simulink model "Sixphase_PMSM_doubleDQ"  (R2023b)
settings: Solver=ode23t  StartTime=0.0  StopTime=0.5  MaxStep=1e-4  RelTol=1e-3  EnableMultiTasking=on
InitFcn:
  | Ts = 1e-6;
undefined symbols (not defined in the file): powergui, sps_lib
libraries: powerlib_extras x7, spsVoltageMeasurementLib x4, spsUniversalBridgeLib x2, spsDCVoltageSourceLib x1
settings Model: Creator=y  LastModifiedBy=Guoguo
settings SolverCC: AlgebraicLoopSolver=TrustRegion
settings DataIOCC: LimitDataPoints=on  SaveFormat=Array  SignalLoggingSaveFormat=ModelDataLogs  ReturnWorkspaceOutputs=off
settings OptimizationCC: ExpressionDepthLimit=2147483647  InitFltsAndDblsToZero=on  LifeSpan=inf
settings DebuggingCC: SaveWithParameterizedLinksMsg=none  UnderspecifiedInitializationDetection=Classic  MergeDetectMultiDrivingBlocksExec=none  SignalResolutionControl=TryResolveAllWithWarning  SolverPrmCheckMsg=warning  MultiTaskDSMMsg=warning  MultiTaskCondExecSysMsg=none  FcnCallInpInsideContextMsg=warning  UnconnectedInputMsg=warning  UnconnectedOutputMsg=warning  UnconnectedLineMsg=warning  StateNameClashWarn=warning  SFUnexpectedBacktrackingDiag=warning  SFNoUnconditionalDefaultTransitionDiag=warning  SFExecutionAtInitializationDiag=none  ArithmeticOperatorsInVariantConditions=warning
settings HardwareCC: ProdBitPerPointer=32  ProdBitPerSizeT=32  ProdBitPerPtrDiffT=32  ProdLargestAtomicFloat=None  ProdIntDivRoundTo=Undefined  ProdEndianess=Unspecified  ProdWordSize=32  ProdHWDeviceType=32-bit Generic
settings ModelReferenceCC: PropagateSignalLabelsOutOfModel=off
settings SFSimCC: SimUseLocalCustomCode=off  CustomCodeUndefinedFunction=UseInterfaceOnly
settings RTWCC: RTWUseLocalCustomCode=off
settings CodeAppCC: StateflowObjectComments=on
settings GRTTargetCC: TargetFcnLib=ansi_tfl_tmw.mat  TargetLangStandard=C89/C90 (ANSI)  CombineOutputUpdateFcns=off  GRTInterface=on
settings ConfigComp: CovMetricSettings=dw  CovSaveCumulativeToWorkspaceVar=on  CovSaveSingleToWorkspaceVar=on  CovExternalEMLEnable=off  CovSFcnEnable=off
settings SimscapeCC: SimscapeNormalizeSystem=off

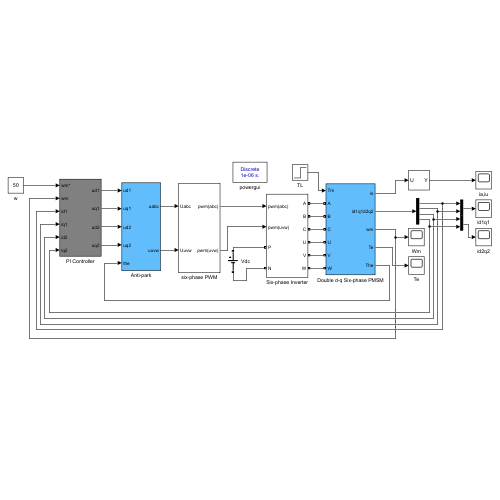
[thumbnail: Simulink's stored preview of the top-level diagram]
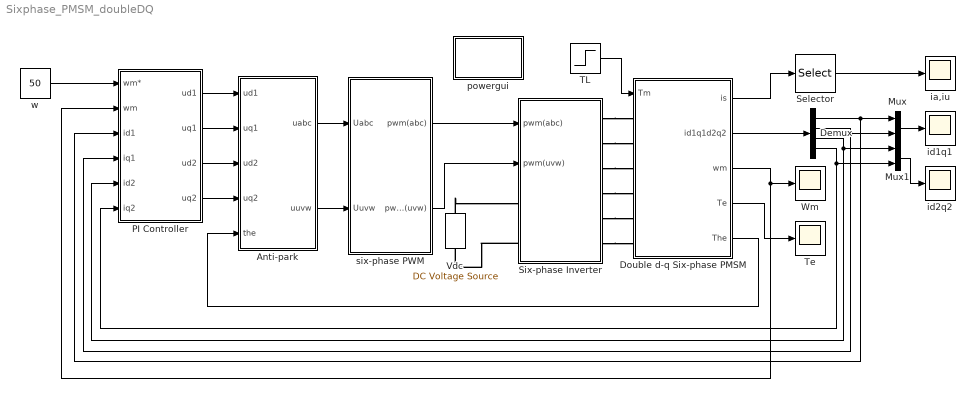
== system Sixphase_PMSM_doubleDQ ==
  Anti-park : Subsystem
  Demux : Demux
  Double d-q Six-phase PMSM : Subsystem  mask{R=1.4, Ld=4.85e-3, Lq=4.85e-3, Ldd=3.15e-3, Lqq=3.15e-3, p=3, Flux=0.68, J=0.015, F=0}
  Mux : Mux  Inputs=2
  Mux1 : Mux  Inputs=2
  PI Controller : Subsystem
  Selector : Selector  InputPortWidth=6  IndexOptions=Index vector (dialog)  Indices=[1 4]  OutputSizes=1
  Six-phase Inverter : Subsystem
  TL : Step  Time=0.2  After=50  SampleTime=0
  Te : Scope
  Vdc : spsDCVoltageSourceLib/DC Voltage Source  Amplitude=300  Measurements=None
  Wm : Scope
  ia,iu : Scope
  id1q1 : Scope
  id2q2 : Scope
  powergui : Subsystem  Priority=1  AncestorBlock=sps_lib/powergui  InitFcn=powergui( 'InitFcn_Callback' , gcb , 0 , [ ] );  mask(PSB option menu block){SimulationMode=Discrete, SampleTime=1e-6, frequency=60, Iterations=50, frequencyindice=0, Pbase=100e6, ErrMax=1e-4, UnitsV=kV, UnitsW=MW, buscounter=0, FunctionMessages=off, echomessages=off, EnableUseOfTLC=off, CurrentSourceSwitches=on, DisableSnubberDevices=off, DisableRonSwitches=off, DisableVfSwitches=off, DisplayEquations=off, AutomaticDiscreteSolvers=off, SolverType=Tustin/Backward Euler (TBE), Interpol=off, ExternalGateDelay=off, methode=off, Ts=100, x0status=blocks, SPID=off, SwTol=0, HookPort=off, NonlinearTolerance=1e-4, nMaxIteration=100, ContinueOnMaxIteration=off, RestoreLinks=warning, ResistiveCurrentMeasurement=off, Frange=[0:2:500], Ylog=off, Xlog=on, ShowGrid=off, save=off, variable=ZData, structure=0, ZoomFFT=off, StartTime=0.0, cycles=1, DisplayStyle=1, fundamental=60, FreqAxis=off, MaxFrequency=1000, frequencyindicesteady=1, RmsSteady=1, display=off}
      mask prompts: SimulationMode "Simulation type:"; SampleTime "Sample time (s):"; frequency "Frequency (Hz):"; Iterations "Max iterations"; frequencyindice "Frequency (Hz)"; Pbase "Base power (VA)"; ErrMax "PQ tolerance (pu)"; UnitsV "Voltage units"; UnitsW "Power units"; buscounter "Load flow bus counter"; FunctionMessages "Disable Specialized Power Systems warnings"; echomessages "Display Specialized Power Systems compilation messages"; EnableUseOfTLC "Use TLC file when in Accelerator Simulation Mode and for code generation"; CurrentSourceSwitches "Disable ideal switching"; DisableSnubberDevices "Disable snubbers in switching devices"; DisableRonSwitches "Disable Ron resistances in switching devices"; DisableVfSwitches "Disable forward voltages in switching devices"; DisplayEquations "Display circuit differential equations"; AutomaticDiscreteSolvers "Automatically handle Discrete solver and Advanced tab solver settings of blocks"; SolverType "Discrete solver"; Interpol "Interpolate switching events"; ExternalGateDelay "Use time-stamped gate signals"; methode "Store switching topologies"; Ts "Buffer size (MBytes):"; x0status "Start simulation with initial electrical states from:"; SPID "Use ideal switching devices"; SwTol "Switch tolerance"; HookPort "Allow multiple powergui blocks"; NonlinearTolerance "Solver tolerance"; nMaxIteration "Maximum number of iterations"; ContinueOnMaxIteration "Continue Simulation if maximum number of iterations is reached"; RestoreLinks "Restore disabled links of Simscape Power Systems ST blocks:"; ResistiveCurrentMeasurement "Use non ideal current measurement blocks (1e-4Ohm internal resistance)"; Frange "Frequency Range"; Ylog "Log impedance"; Xlog "log Frequency"; ShowGrid "grid"; save "Save Data To Workspace"; variable "Variable Name"; structure "Structure Name (PSBFFTSCOPE)"; ZoomFFT "ZoomFFT (PSBFFTSCOPE)"; StartTime "Start Time (PSBFFTSCOPE)"; cycles "Cycles (PSBFFTSCOPE)"; DisplayStyle "Display style (PSBFFTSCOPE)"; fundamental "Fundamental (PSBFFTSCOPE)"; FreqAxis "Frequency Axis (PSBFFTSCOPE)"; MaxFrequency "Max Frequency (PSBFFTSCOPE)"; frequencyindicesteady "Frequency indice (STEADYSTATE)"; RmsSteady "RMS display (STEADYSTATE)"; display "Display Results"
      mask help: Set simulation type, simulation parameters, and preferences.
      mask init:
      | dispMessage = '';
      | dispMessage = powergui('MaskInitialization',gcb,SimulationMode,SampleTime);
      settings: LibrarySourceBlock=sps_lib/powergui  PreSaveFcn=powergui( 'PreSaveFcn_Callback' , gcb , [ ] , [ ] );  OpenFcn=sps_rtmsupport('OpenFcn',gcbh)
      mask Help: helpview(psbhelp)
      mask TypeOptions SimulationMode: Continuous | Discrete | Phasor | Discrete phasor
      mask Callback SimulationMode: powergui('SimulationType',[],[],gcb);
      mask TypeOptions UnitsV: V | kV
      mask TypeOptions UnitsW: W | kW | MW
      mask Callback CurrentSourceSwitches: powergui('SimulationType',[],[],gcb);
      mask Callback AutomaticDiscreteSolvers: powergui('SimulationType',[],[],gcb);
      mask TypeOptions SolverType: Tustin/Backward Euler (TBE) | Tustin | Backward Euler
      mask Callback SolverType: powergui('SimulationType',[],[],gcb);
      mask Callback Interpol: powergui('SimulationType',[],[],gcb);
      mask Callback ExternalGateDelay: powergui('SimulationType',[],[],gcb);
      mask Callback methode: powergui('SimulationType',[],[],gcb);
      mask TypeOptions x0status: blocks | steady | zero
      mask TypeOptions RestoreLinks: yes | warning | no
      mask Callback display: sps_rtmsupport('parametereditingmodes',gcbh) % Will be executed last in parameter callbacks to ensure mask enable consistency
      mask DialogControl SolverTab Prompt: Solver
      mask DialogControl AutoSolverNote Prompt: The Simulation type parameter is governed by Simulink. To access the Powergui solver settings, unselect auto (Automatic solver selection) solver in the Simulink solver options.
      mask DialogControl Apps Prompt: Apps
      mask DialogControl StateAnalyzer Prompt: Measurements and States Analyzer
      mask DialogControl StateAnalyzer Callback: powerStates(bdroot(gcb))
      mask DialogControl LineParameterCalculator Prompt: Line Parameter Calculator
      mask DialogControl LineParameterCalculator Callback:
      | close_system(gcb)
      | powerLineParameters
      mask DialogControl CableParameterCalculator Prompt: Cable Parameter Calculator
      mask DialogControl CableParameterCalculator Callback:
      | close_system(gcb)
      | powerCableParameters
      mask DialogControl LineDecoupler Prompt: Line Decoupler
      mask DialogControl LineDecoupler Tooltip: Click to replace selected Distributed Parameters Line blocks with Decoupling Line blocks
      mask DialogControl LineDecoupler Callback:
      | close_system(gcb);
      | DecouplingLineReplace(gcs)
      mask DialogControl LoadFlowAnalyzer Prompt: Load Flow Analyzer
      mask DialogControl LoadFlowAnalyzer Callback:
      | close_system(gcb)
      | powerLoadFlow
      mask DialogControl LoadFlowParameters Prompt: Load Flow Parameters
      mask DialogControl ImpedanceCalculator Prompt: Impedance Calculator
      mask DialogControl ImpedanceCalculator Callback:
      | close_system(gcb);
      | powerImpedance(bdroot(gcs));
      mask DialogControl FFTAnalyzer Prompt: FFT Analyzer
      mask DialogControl FFTAnalyzer Callback:
      | close_system(gcb)
      | power_fftscope(bdroot(gcb),gcb)
      mask DialogControl LinearSystemAnalyzer Prompt: Linear System Analyzer
      mask DialogControl LinearSystemAnalyzer Callback:
      | close_system(gcb)
      | power_ltiview(bdroot(gcb))
      mask DialogControl HysteresisDesigner Prompt: Hysteresis Designer
      mask DialogControl HysteresisDesigner Callback:
      | close_system(gcb)
      | powerHysteresis('hysteresis.mat')
      mask DialogControl BlockCustomizer Prompt: Block Customizer
      mask DialogControl BlockCustomizer Callback:
      | close_system(gcb);
      | power_customize;
      mask DialogControl ReportGenerator Prompt: Report Generator
      mask DialogControl ReportGenerator Callback:
      | close_system(gcb)
      | power_report(bdroot(gcb))
      mask DialogControl obsolete Prompt: ...
      mask DialogControl MachineInitialization Prompt: Machine Initialization
      mask DialogControl MachineInitialization Callback:
      | close_system(gcb)
      | powericon('machineInitTool',bdroot(gcb),gcb)
      mask DialogControl Preferences Prompt: Preferences
      mask DialogControl Solver Prompt: Solver
      mask DialogControl SolverDetails Prompt: Solver details for nonlinear elements
      mask Display: color('blue'),disp(dispMessage)
  six-phase PWM : Subsystem
  w : Constant  Value=50
  wires:
  Double d-q Six-phase PMSM/2(id1q1d2q2) -> Demux/1
  Demux/1 -> Mux/1, PI Controller/3(id1)
  Demux/2 -> Mux/2, PI Controller/4(iq1)
  Demux/3 -> Mux1/1, PI Controller/5(id2)
  Demux/4 -> Mux1/2, PI Controller/6(iq2)
  Double d-q Six-phase PMSM/5(The) -> Anti-park/5(the)
  Double d-q Six-phase PMSM/3(wm) -> Wm/1, PI Controller/2(wm)
  w/1 -> PI Controller/1(wm*)
  PI Controller/1(ud1) -> Anti-park/1(ud1)
  PI Controller/2(uq1) -> Anti-park/2(uq1)
  PI Controller/3(ud2) -> Anti-park/3(ud2)
  PI Controller/4(uq2) -> Anti-park/4(uq2)
  TL/1 -> Double d-q Six-phase PMSM/1(Tm)
  six-phase PWM/1(pwm(abc)) -> Six-phase Inverter/1(pwm(abc))
  six-phase PWM/2(pwm(uvw)) -> Six-phase Inverter/2(pwm(uvw))
  Anti-park/2(uuvw) -> six-phase PWM/2(Uuvw)
  Anti-park/1(uabc) -> six-phase PWM/1(Uabc)
  Selector/1 -> ia,iu/1
  Double d-q Six-phase PMSM/1(is) -> Selector/1
  Mux/1 -> id1q1/1
  Mux1/1 -> id2q2/1
  Double d-q Six-phase PMSM/4(Te) -> Te/1
  connections:
  Vdc/RConn1 -- Six-phase Inverter/LConn1
  Six-phase Inverter/LConn2 -- Vdc/LConn1
  Six-phase Inverter/RConn1 -- Double d-q Six-phase PMSM/LConn1
  Six-phase Inverter/RConn2 -- Double d-q Six-phase PMSM/LConn2
  Six-phase Inverter/RConn3 -- Double d-q Six-phase PMSM/LConn3
  Six-phase Inverter/RConn4 -- Double d-q Six-phase PMSM/LConn4
  Six-phase Inverter/RConn5 -- Double d-q Six-phase PMSM/LConn5
  Six-phase Inverter/RConn6 -- Double d-q Six-phase PMSM/LConn6

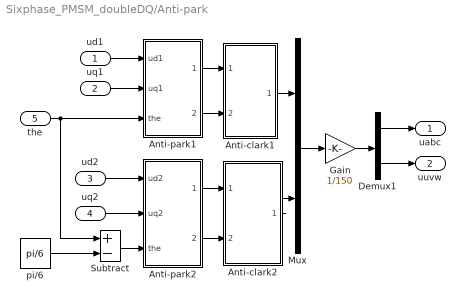
== system Sixphase_PMSM_doubleDQ/Anti-park ==
  ud1 : Inport
  uq1 : Inport  Port=2
  ud2 : Inport  Port=3
  uq2 : Inport  Port=4
  the : Inport  Port=5
  Anti-clark1 : Subsystem
  Anti-clark2 : Subsystem
  Anti-park1 : Subsystem
  Anti-park2 : Subsystem
  Demux1 : Demux  Outputs=2
  Gain : Gain  Gain=1/150
  Mux : Mux  Inputs=2
  Subtract : Sum  Inputs=+-
  pi/6 : Constant  Value=pi/6
  uabc : Outport
  uuvw : Outport  Port=2
  wires:
  Anti-clark1/1(uabc) -> Mux/1
  Anti-clark2/1(uuvw) -> Mux/2
  Mux/1 -> Gain/1
  Anti-park1/1(ualpha1) -> Anti-clark1/1(ualpha)
  Anti-park1/2(ubeta1) -> Anti-clark1/2(ubeta)
  Anti-park2/1(ualpha2) -> Anti-clark2/1(ualpha)
  Anti-park2/2(ubeta2) -> Anti-clark2/2(ubeta)
  ud1/1 -> Anti-park1/1(ud1)
  uq1/1 -> Anti-park1/2(uq1)
  ud2/1 -> Anti-park2/1(ud2)
  uq2/1 -> Anti-park2/2(uq2)
  Gain/1 -> Demux1/1
  Demux1/1 -> uabc/1
  Demux1/2 -> uuvw/1
  the/1 -> Subtract/1, Anti-park1/3(the)
  Subtract/1 -> Anti-park2/3(the)
  pi/6/1 -> Subtract/2

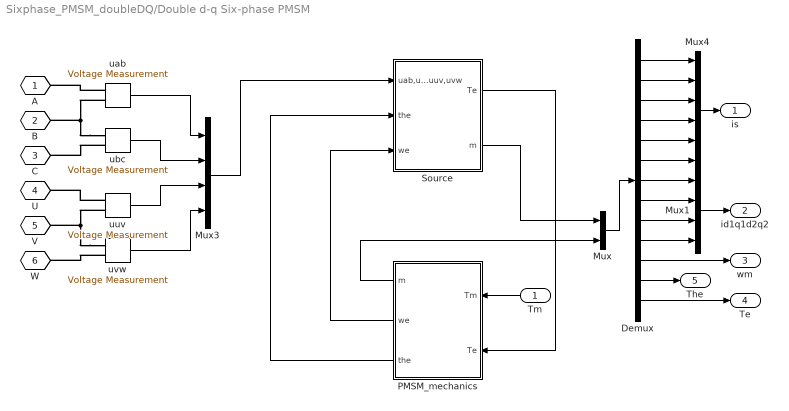
== system Sixphase_PMSM_doubleDQ/Double d-q Six-phase PMSM ==
  Tm : Inport
  Demux : Demux  Outputs=13
  Mux : Mux  Inputs=2
  Mux1 : Mux
  Mux3 : Mux
  Mux4 : Mux  Inputs=6
  PMSM_mechanics : Subsystem
  Source : Subsystem
  uab : spsVoltageMeasurementLib/Voltage Measurement  PhasorSimulation=off  OutputType=Complex  PSBequivalent=0
  ubc : spsVoltageMeasurementLib/Voltage Measurement  PhasorSimulation=off  OutputType=Complex  PSBequivalent=0
  uuv : spsVoltageMeasurementLib/Voltage Measurement  PhasorSimulation=off  OutputType=Complex  PSBequivalent=0
  uvw : spsVoltageMeasurementLib/Voltage Measurement  PhasorSimulation=off  OutputType=Complex  PSBequivalent=0
  A : PMIOPort  Tag=PMCPort  Side=Left
  B : PMIOPort  Tag=PMCPort  Port=2  Side=Left
  C : PMIOPort  Tag=PMCPort  Port=3  Side=Left
  U : PMIOPort  Tag=PMCPort  Port=4  Side=Left
  V : PMIOPort  Tag=PMCPort  Port=5  Side=Left
  W : PMIOPort  Tag=PMCPort  Port=6  Side=Left
  is : Outport
  id1q1d2q2 : Outport  Port=2
  wm : Outport  Port=3
  Te : Outport  Port=4
  The : Outport  Port=5
  wires:
  Tm/1 -> PMSM_mechanics/1(Tm)
  Source/1(Te) -> PMSM_mechanics/2(Te)
  PMSM_mechanics/3(the) -> Source/2(the)
  PMSM_mechanics/2(we) -> Source/3(we)
  PMSM_mechanics/1(m) -> Mux/2
  Source/2(m) -> Mux/1
  Mux/1 -> Demux/1
  Demux/1 -> Mux4/1
  Demux/2 -> Mux4/2
  Demux/3 -> Mux4/3
  Demux/4 -> Mux4/4
  Demux/5 -> Mux4/5
  Demux/6 -> Mux4/6
  Mux4/1 -> is/1
  Demux/7 -> Mux1/1
  Demux/8 -> Mux1/2
  Demux/9 -> Mux1/3
  Demux/10 -> Mux1/4
  Mux1/1 -> id1q1d2q2/1
  Mux3/1 -> Source/1(uab,ubc,uuv,uvw)
  uab/1 -> Mux3/1
  ubc/1 -> Mux3/2
  uuv/1 -> Mux3/3
  uvw/1 -> Mux3/4
  Demux/11 -> wm/1
  Demux/12 -> The/1
  Demux/13 -> Te/1
  connections:
  ubc/LConn1 -- uab/LConn2 -- B/RConn1
  uvw/LConn1 -- uuv/LConn2 -- V/RConn1
  uvw/LConn2 -- W/RConn1
  uab/LConn1 -- A/RConn1
  ubc/LConn2 -- C/RConn1
  uuv/LConn1 -- U/RConn1

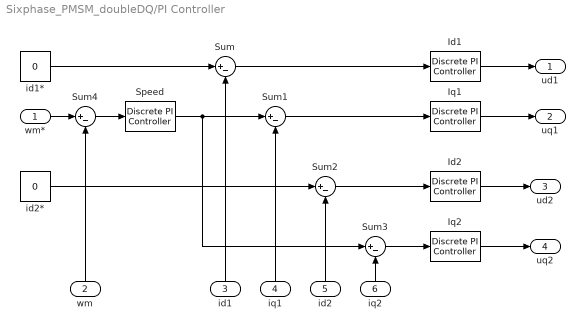
== system Sixphase_PMSM_doubleDQ/PI Controller ==
  wm* : Inport
  wm : Inport  Port=2
  id1 : Inport  Port=3
  iq1 : Inport  Port=4
  id2 : Inport  Port=5
  iq2 : Inport  Port=6
  Id1 : powerlib_extras/Discrete  Control Blocks/Discrete PI Controller  Kp=0.008*1200  Ki=1.4*1200  Par_Limits=[400 -400]  Init=0  Ts=Ts
  Id2 : powerlib_extras/Discrete  Control Blocks/Discrete PI Controller  Kp=0.008*1200  Ki=1.4*1200  Par_Limits=[400 -400]  Init=0  Ts=Ts
  Iq1 : powerlib_extras/Discrete  Control Blocks/Discrete PI Controller  Kp=0.008*1200  Ki=1.4*1200  Par_Limits=[400 -400]  Init=0  Ts=Ts
  Iq2 : powerlib_extras/Discrete  Control Blocks/Discrete PI Controller  Kp=0.008*1200  Ki=1.4*1200  Par_Limits=[400 -400]  Init=0  Ts=Ts
  Speed : powerlib_extras/Discrete  Control Blocks/Discrete PI Controller  Kp=1  Ki=80  Par_Limits=[25 -25]  Init=0  Ts=Ts
  Sum{,1..4} (5 alike) : Sum  Inputs=|+-
  id1* : Constant  Value=0
  id2* : Constant  Value=0
  ud1 : Outport
  uq1 : Outport  Port=2
  ud2 : Outport  Port=3
  uq2 : Outport  Port=4
  wires:
  Sum3/1 -> Iq2/1
  Sum2/1 -> Id2/1
  Sum1/1 -> Iq1/1
  Sum/1 -> Id1/1
  Sum4/1 -> Speed/1
  Speed/1 -> Sum1/1, Sum3/1
  id1/1 -> Sum/2
  iq1/1 -> Sum1/2
  wm/1 -> Sum4/2
  id2/1 -> Sum2/2
  iq2/1 -> Sum3/2
  Id1/1 -> ud1/1
  id1*/1 -> Sum/1
  wm*/1 -> Sum4/1
  Iq1/1 -> uq1/1
  Id2/1 -> ud2/1
  id2*/1 -> Sum2/1
  Iq2/1 -> uq2/1

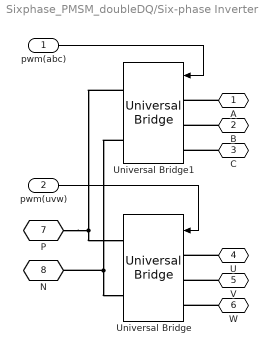
== system Sixphase_PMSM_doubleDQ/Six-phase Inverter ==
  pwm(abc) : Inport
  pwm(uvw) : Inport  Port=2
  Universal Bridge : spsUniversalBridgeLib/Universal Bridge  Arms=3  SnubberResistance=1e5  SnubberCapacitance=inf  Device=IGBT / Diodes  Ron=1e-3  Lon=0  ForwardVoltages="[  0  0  ]"  ForwardVoltage=0  GTOparameters=[ 10e-6 , 20e-6 ]  IGBTparameters=[ 1e-6 , 2e-6 ]  Measurements=None  Measurements_2=None  converterType=Rectifier
  Universal Bridge1 : spsUniversalBridgeLib/Universal Bridge  Arms=3  SnubberResistance=1e5  SnubberCapacitance=inf  Device=IGBT / Diodes  Ron=1e-3  Lon=0  ForwardVoltages="[  0  0  ]"  ForwardVoltage=0  GTOparameters=[ 10e-6 , 20e-6 ]  IGBTparameters=[ 1e-6 , 2e-6 ]  Measurements=None  Measurements_2=None  converterType=Rectifier
  A : PMIOPort  Side=Right
  B : PMIOPort  Port=2  Side=Right
  C : PMIOPort  Port=3  Side=Right
  U : PMIOPort  Port=4  Side=Right
  V : PMIOPort  Port=5  Side=Right
  W : PMIOPort  Port=6  Side=Right
  P : PMIOPort  Port=7  Side=Left
  N : PMIOPort  Port=8  Side=Left
  wires:
  pwm(abc)/1 -> Universal Bridge1/1
  pwm(uvw)/1 -> Universal Bridge/1
  connections:
  A/RConn1 -- Universal Bridge1/LConn1
  C/RConn1 -- Universal Bridge1/LConn3
  W/RConn1 -- Universal Bridge/LConn3
  B/RConn1 -- Universal Bridge1/LConn2
  U/RConn1 -- Universal Bridge/LConn1
  V/RConn1 -- Universal Bridge/LConn2
  Universal Bridge1/RConn1 -- P/RConn1 -- Universal Bridge/RConn1
  Universal Bridge1/RConn2 -- N/RConn1 -- Universal Bridge/RConn2

== system Sixphase_PMSM_doubleDQ/powergui ==
  note: Graphical user interface for the analysis of
      | Simscape Power Systems (Specialized Technology) circuits.
      | Place the Powergui block in the top-level of your model and double-click
      | on it to open the GUI.
  EquivalentModel1 : Subsystem
      mask init:
      | S  = GetDataForEquivalentModel('Discrete',gcbh);
      mask Display:
      | color('red')
      | disp('EQUIVALENT CIRCUIT\nDiscrete')
  Ground : Ground
  Terminator : Terminator
  wires:
  Ground/1 -> Terminator/1

== system Sixphase_PMSM_doubleDQ/six-phase PWM ==
  Uabc : Inport
  Uuvw : Inport  Port=2
  Discrete PWM Generator : powerlib_extras/Discrete  Control Blocks/Discrete PWM Generator  GeneratorMode="3-arm  bridge (6 pulses)"  Fc=10000  Ts=1e-6  Internal=off  mIndex=0.4  Freq=60  Phase=0
  Discrete PWM Generator1 : powerlib_extras/Discrete  Control Blocks/Discrete PWM Generator  GeneratorMode="3-arm  bridge (6 pulses)"  Fc=10000  Ts=1e-6  Internal=off  mIndex=0.4  Freq=60  Phase=0
  pwm(abc) : Outport
  pwm(uvw) : Outport  Port=2
  wires:
  Uabc/1 -> Discrete PWM Generator/1
  Discrete PWM Generator1/1 -> pwm(uvw)/1
  Uuvw/1 -> Discrete PWM Generator1/1
  Discrete PWM Generator/1 -> pwm(abc)/1

== system Sixphase_PMSM_doubleDQ/Anti-park/Anti-clark1 ==
  ualpha : Inport
  ubeta : Inport  Port=2
  Fcn : Fcn  Expr=u[1]
  Fcn1 : Fcn  Expr=-1/2*u[1]+sqrt(3)/2*u[2]
  Fcn2 : Fcn  Expr=-1/2*u[1]-sqrt(3)/2*u[2]
  Mux : Mux  Inputs=3
  Mux1 : Mux  Inputs=2
  uabc : Outport
  wires:
  Fcn/1 -> Mux/1
  Fcn1/1 -> Mux/2
  Fcn2/1 -> Mux/3
  Mux/1 -> uabc/1
  Mux1/1 -> Fcn1/1, Fcn/1, Fcn2/1
  ubeta/1 -> Mux1/2
  ualpha/1 -> Mux1/1

== system Sixphase_PMSM_doubleDQ/Anti-park/Anti-clark2 ==
  ualpha : Inport
  ubeta : Inport  Port=2
  Fcn : Fcn  Expr=u[1]
  Fcn1 : Fcn  Expr=-1/2*u[1]+sqrt(3)/2*u[2]
  Fcn2 : Fcn  Expr=-1/2*u[1]-sqrt(3)/2*u[2]
  Mux : Mux  Inputs=3
  Mux1 : Mux  Inputs=2
  uuvw : Outport
  wires:
  Fcn/1 -> Mux/1
  Fcn1/1 -> Mux/2
  Fcn2/1 -> Mux/3
  Mux/1 -> uuvw/1
  Mux1/1 -> Fcn1/1, Fcn/1, Fcn2/1
  ubeta/1 -> Mux1/2
  ualpha/1 -> Mux1/1

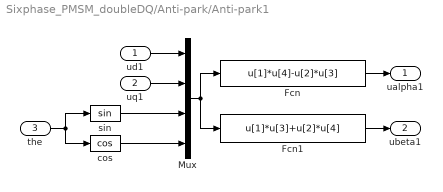
== system Sixphase_PMSM_doubleDQ/Anti-park/Anti-park1 ==
  ud1 : Inport
  uq1 : Inport  Port=2
  the : Inport  Port=3
  Fcn : Fcn  Expr=u[1]*u[4]-u[2]*u[3]
  Fcn1 : Fcn  Expr=u[1]*u[3]+u[2]*u[4]
  Mux : Mux
  cos : Trigonometry  Operator=cos
  sin : Trigonometry
  ualpha1 : Outport
  ubeta1 : Outport  Port=2
  wires:
  ud1/1 -> Mux/1
  uq1/1 -> Mux/2
  Mux/1 -> Fcn1/1, Fcn/1
  sin/1 -> Mux/3
  cos/1 -> Mux/4
  the/1 -> sin/1, cos/1
  Fcn/1 -> ualpha1/1
  Fcn1/1 -> ubeta1/1

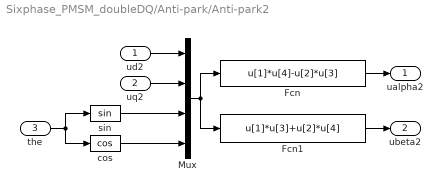
== system Sixphase_PMSM_doubleDQ/Anti-park/Anti-park2 ==
  ud2 : Inport
  uq2 : Inport  Port=2
  the : Inport  Port=3
  Fcn : Fcn  Expr=u[1]*u[4]-u[2]*u[3]
  Fcn1 : Fcn  Expr=u[1]*u[3]+u[2]*u[4]
  Mux : Mux
  cos : Trigonometry  Operator=cos
  sin : Trigonometry
  ualpha2 : Outport
  ubeta2 : Outport  Port=2
  wires:
  ud2/1 -> Mux/1
  uq2/1 -> Mux/2
  Mux/1 -> Fcn1/1, Fcn/1
  sin/1 -> Mux/3
  cos/1 -> Mux/4
  the/1 -> sin/1, cos/1
  Fcn/1 -> ualpha2/1
  Fcn1/1 -> ubeta2/1

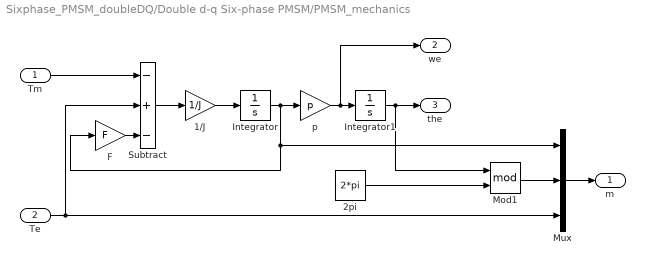
== system Sixphase_PMSM_doubleDQ/Double d-q Six-phase PMSM/PMSM_mechanics ==
  Tm : Inport
  Te : Inport  Port=2
  1/J : Gain  Gain=1/J
  2pi : Constant  Value=2*pi
  F : Gain  Gain=F
  Integrator : Integrator
  Integrator1 : Integrator
  Mod1 : Math  Operator=mod  SignedPower=on
  Mux : Mux  Inputs=3
  Subtract : Sum  Inputs=-+-
  p : Gain  Gain=p
  m : Outport
  we : Outport  Port=2
  the : Outport  Port=3
  wires:
  Tm/1 -> Subtract/1
  Te/1 -> Mux/3, Subtract/2
  Subtract/1 -> 1/J/1
  1/J/1 -> Integrator/1
  Integrator/1 -> p/1, F/1, Mux/1
  F/1 -> Subtract/3
  p/1 -> Integrator1/1, we/1
  Mux/1 -> m/1
  Integrator1/1 -> Mod1/1, the/1
  Mod1/1 -> Mux/2
  2pi/1 -> Mod1/2

== system Sixphase_PMSM_doubleDQ/Double d-q Six-phase PMSM/Source ==
  uab,ubc,uuv,uvw : Inport
  the : Inport  Port=2
  we : Inport  Port=3
  Mux : Mux  Inputs=2
  abcuvw->d1q1d2q2 : Subsystem
  d1q1d2q2->abcuvw : Subsystem
  id1,iq1,id2,iq2 : Subsystem
  Te : Outport
  m : Outport  Port=2
  wires:
  abcuvw->d1q1d2q2/2(ud1,uq1,ud2,uq2) -> id1,iq1,id2,iq2/1(ud1,uq1,ud2,uq2)
  id1,iq1,id2,iq2/1(id1,i1,id2,iq2) -> d1q1d2q2->abcuvw/2(id1,iq1,id2,iq2), Mux/2
  abcuvw->d1q1d2q2/1(s1,c1,s2,c2) -> d1q1d2q2->abcuvw/1(s1,c1,s2,c2)
  uab,ubc,uuv,uvw/1 -> abcuvw->d1q1d2q2/1(uab,ubc,uuv,uvw)
  d1q1d2q2->abcuvw/1(is) -> Mux/1
  the/1 -> abcuvw->d1q1d2q2/2(the)
  we/1 -> id1,iq1,id2,iq2/2(we)
  id1,iq1,id2,iq2/2(Te) -> Te/1
  Mux/1 -> m/1

== system Sixphase_PMSM_doubleDQ/powergui/EquivalentModel1 ==
  Gates : Subsystem
  Sources : Subsystem
  State-Space : S-Function  FunctionName=sfun_spssw_discc  Parameters=S.Ts,S.A, S.B, S.C, S.D, S.x0, S.EnableUseOfTLC,S.SwitchResistance ,S.SwitchType, S.SwitchGateInitialValue, S.OutputsToResetToZero, S.TBEON,S.SaveMatrices,S.BufferSize  SFunctionDeploymentMode=off  EnableBusSupport=off
  Status : Subsystem
  Yout : Subsystem
  wires:
  State-Space/1 -> Yout/1(v,i)
  State-Space/2 -> Status/1(status)
  Sources/1(u) -> State-Space/1
  Gates/1(gates) -> State-Space/2

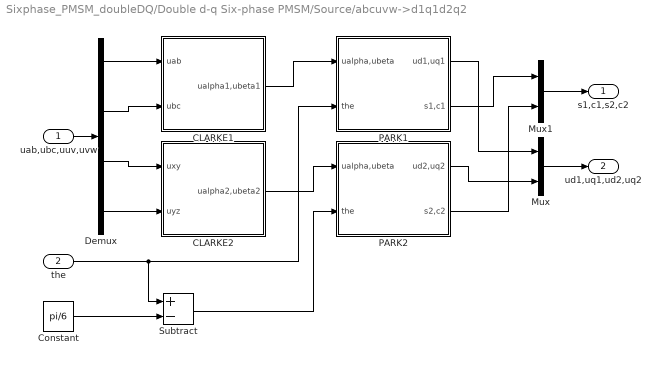
== system Sixphase_PMSM_doubleDQ/Double d-q Six-phase PMSM/Source/abcuvw->d1q1d2q2 ==
  uab,ubc,uuv,uvw : Inport
  the : Inport  Port=2
  CLARKE1 : Subsystem
  CLARKE2 : Subsystem
  Constant : Constant  Value=pi/6
  Demux : Demux
  Mux : Mux  Inputs=2
  Mux1 : Mux  Inputs=2
  PARK1 : Subsystem
  PARK2 : Subsystem
  Subtract : Sum  Inputs=+-
  s1,c1,s2,c2 : Outport
  ud1,uq1,ud2,uq2 : Outport  Port=2
  wires:
  the/1 -> Subtract/1, PARK1/2(the)
  Constant/1 -> Subtract/2
  Subtract/1 -> PARK2/2(the)
  CLARKE1/1(ualpha1,ubeta1) -> PARK1/1(ualpha,ubeta)
  CLARKE2/1(ualpha2,ubeta2) -> PARK2/1(ualpha,ubeta)
  PARK1/2(s1,c1) -> Mux1/1
  PARK1/1(ud1,uq1) -> Mux/1
  PARK2/1(ud2,uq2) -> Mux/2
  PARK2/2(s2,c2) -> Mux1/2
  Mux1/1 -> s1,c1,s2,c2/1
  Mux/1 -> ud1,uq1,ud2,uq2/1
  uab,ubc,uuv,uvw/1 -> Demux/1
  Demux/1 -> CLARKE1/1(uab)
  Demux/2 -> CLARKE1/2(ubc)
  Demux/3 -> CLARKE2/1(uxy)
  Demux/4 -> CLARKE2/2(uyz)

== system Sixphase_PMSM_doubleDQ/Double d-q Six-phase PMSM/Source/d1q1d2q2->abcuvw ==
  s1,c1,s2,c2 : Inport
  id1,iq1,id2,iq2 : Inport  Port=2
  Demux : Demux  Outputs=2
  Demux1 : Demux  Outputs=2
  ICLARKE1 : Subsystem
  ICLARKE2 : Subsystem
  IPARK : Subsystem
  IPARK1 : Subsystem
  Mux : Mux  Inputs=2
  is : Outport
  wires:
  IPARK/1(ialpha1,ibeta1) -> ICLARKE1/1(ialpha1.ibeta1)
  IPARK1/1(ialpha2,ibeta2) -> ICLARKE2/1(ialpha2.ibeta2)
  ICLARKE1/1(iabc) -> Mux/1
  ICLARKE2/1(ixyz) -> Mux/2
  Mux/1 -> is/1
  id1,iq1,id2,iq2/1 -> Demux1/1
  s1,c1,s2,c2/1 -> Demux/1
  Demux1/1 -> IPARK/1(id1,iq1)
  Demux1/2 -> IPARK1/1(id2,iq2)
  Demux/1 -> IPARK/2(s1,c1)
  Demux/2 -> IPARK1/2(s2,c2)

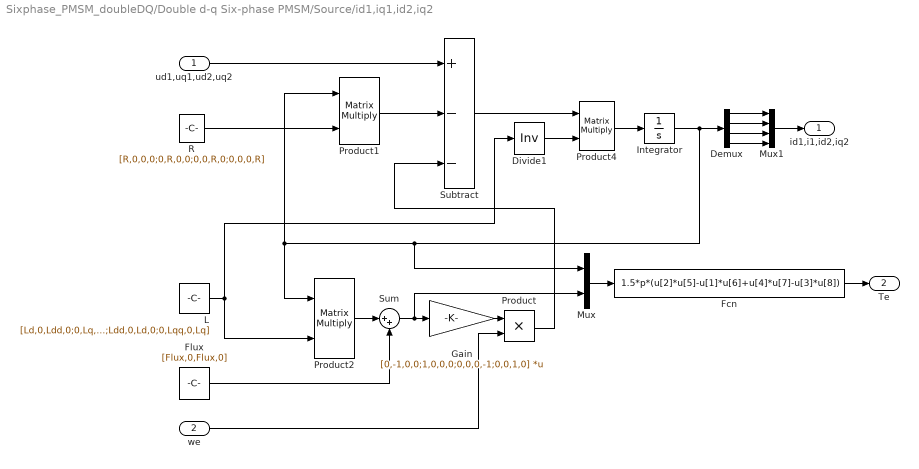
== system Sixphase_PMSM_doubleDQ/Double d-q Six-phase PMSM/Source/id1,iq1,id2,iq2 ==
  ud1,uq1,ud2,uq2 : Inport
  we : Inport  Port=2
  Demux : Demux
  Divide1 : Product  Inputs=/  Multiplication=Matrix(*)
  Fcn : Fcn  Expr=1.5*p*(u[2]*u[5]-u[1]*u[6]+u[4]*u[7]-u[3]*u[8])
  Flux : Constant  Value=[Flux,0,Flux,0]
  Gain : Gain  Gain=[0,-1,0,0;1,0,0,0;0,0,0,-1;0,0,1,0]  Multiplication=Matrix(K*u) (u vector)
  Integrator : Integrator
  L : Constant  Value=[Ld,0,Ldd,0;0,Lq,0,Lqq;Ldd,0,Ld,0;0,Lqq,0,Lq]
  Mux : Mux  Inputs=2
  Mux1 : Mux
  Product : Product  RndMeth=Zero
  Product1 : Product  Multiplication=Matrix(*)  RndMeth=Zero
  Product2 : Product  Multiplication=Matrix(*)  RndMeth=Zero
  Product4 : Product  Multiplication=Matrix(*)  RndMeth=Zero
  R : Constant  Value=[R,0,0,0;0,R,0,0;0,0,R,0;0,0,0,R]
  Subtract : Sum  Inputs=+--
  Sum : Sum  Inputs=|++
  id1,i1,id2,iq2 : Outport
  Te : Outport  Port=2
  wires:
  Integrator/1 -> Mux/1, Product1/1, Product2/1, Demux/1
  ud1,uq1,ud2,uq2/1 -> Subtract/1
  L/1 -> Product2/2, Divide1/1
  Product2/1 -> Sum/1
  Flux/1 -> Sum/2
  Sum/1 -> Gain/1, Mux/2
  Gain/1 -> Product/1
  Product1/1 -> Subtract/2
  Product/1 -> Subtract/3
  Product4/1 -> Integrator/1
  Subtract/1 -> Product4/1
  Divide1/1 -> Product4/2
  R/1 -> Product1/2
  we/1 -> Product/2
  Mux/1 -> Fcn/1
  Fcn/1 -> Te/1
  Mux1/1 -> id1,i1,id2,iq2/1
  Demux/1 -> Mux1/1
  Demux/2 -> Mux1/2
  Demux/3 -> Mux1/3
  Demux/4 -> Mux1/4

== system Sixphase_PMSM_doubleDQ/powergui/EquivalentModel1/Gates ==
  Mux : Mux  Inputs=[6 6]
  gates : Outport  VectorParamsAs1DForOutWhenUnconnected=off
  wires:
  Mux/1 -> gates/1
  [T64_6062_6590770816664] -> Mux/1
  [T63_6013_6618727160599] -> Mux/2

== system Sixphase_PMSM_doubleDQ/powergui/EquivalentModel1/Sources ==
  Mux : Mux  Inputs=[6 6 1]
  u : Outport  VectorParamsAs1DForOutWhenUnconnected=off
  wires:
  Mux/1 -> u/1
  [T65_6024_5505210402678] -> Mux/1
  [T64_5975_5558994414286] -> Mux/2
  [T31_2916_1422661067032] -> Mux/3

== system Sixphase_PMSM_doubleDQ/powergui/EquivalentModel1/Status ==
  status : Inport
  Demux : Demux  Outputs=[6 6]
  tag scope: T65_6248_7384193253303=global, T66_6297_7395558894480=global
  wires:
  status/1 -> Demux/1
  Demux/1 -> [T66_6297_7395558894480]
  Demux/2 -> [T65_6248_7384193253303]

== system Sixphase_PMSM_doubleDQ/powergui/EquivalentModel1/Yout ==
  v,i : Inport
  Demux : Demux  Outputs=[6 6 1 1 1 1]
  tag scope: T59_5394_5703294232683=global, T59_5396_5717258194752=global, T59_5434_6038814275815=global, T59_5436_6058698322279=global, T66_6347_7512127218014=global, T67_6396_7536176317992=global
  wires:
  v,i/1 -> Demux/1
  Demux/1 -> [T67_6396_7536176317992]
  Demux/2 -> [T66_6347_7512127218014]
  Demux/3 -> [T59_5394_5703294232683]
  Demux/4 -> [T59_5396_5717258194752]
  Demux/5 -> [T59_5434_6038814275815]
  Demux/6 -> [T59_5436_6058698322279]

== system Sixphase_PMSM_doubleDQ/Double d-q Six-phase PMSM/Source/abcuvw->d1q1d2q2/CLARKE1 ==
  uab : Inport
  ubc : Inport  Port=2
  Fcn : Fcn  Expr=(2*u[1]+u[2])/3
  Fcn1 : Fcn  Expr=sqrt(3)*u[2]/3
  Mux : Mux  Inputs=2
  Mux1 : Mux  Inputs=2
  ualpha1,ubeta1 : Outport
  wires:
  uab/1 -> Mux/1
  Mux/1 -> Fcn/1, Fcn1/1
  ubc/1 -> Mux/2
  Mux1/1 -> ualpha1,ubeta1/1
  Fcn/1 -> Mux1/1
  Fcn1/1 -> Mux1/2

== system Sixphase_PMSM_doubleDQ/Double d-q Six-phase PMSM/Source/abcuvw->d1q1d2q2/CLARKE2 ==
  uxy : Inport
  uyz : Inport  Port=2
  Fcn : Fcn  Expr=(2*u[1]+u[2])/3
  Fcn1 : Fcn  Expr=sqrt(3)*u[2]/3
  Mux : Mux  Inputs=2
  Mux1 : Mux  Inputs=2
  ualpha2,ubeta2 : Outport
  wires:
  uxy/1 -> Mux/1
  Mux/1 -> Fcn/1, Fcn1/1
  uyz/1 -> Mux/2
  Mux1/1 -> ualpha2,ubeta2/1
  Fcn/1 -> Mux1/1
  Fcn1/1 -> Mux1/2

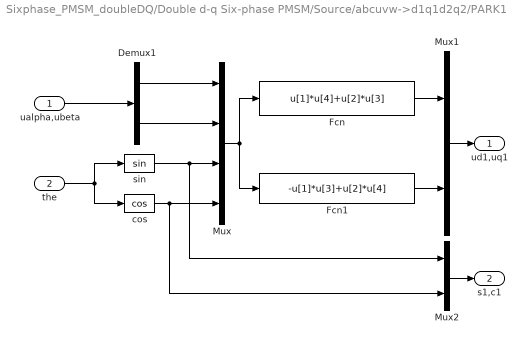
== system Sixphase_PMSM_doubleDQ/Double d-q Six-phase PMSM/Source/abcuvw->d1q1d2q2/PARK1 ==
  ualpha,ubeta : Inport
  the : Inport  Port=2
  Demux1 : Demux  Outputs=2
  Fcn : Fcn  Expr=u[1]*u[4]+u[2]*u[3]
  Fcn1 : Fcn  Expr=-u[1]*u[3]+u[2]*u[4]
  Mux : Mux
  Mux1 : Mux  Inputs=2
  Mux2 : Mux  Inputs=2
  cos : Trigonometry  Operator=cos
  sin : Trigonometry
  ud1,uq1 : Outport
  s1,c1 : Outport  Port=2
  wires:
  Mux/1 -> Fcn/1, Fcn1/1
  ualpha,ubeta/1 -> Demux1/1
  Demux1/1 -> Mux/1
  Demux1/2 -> Mux/2
  sin/1 -> Mux/3, Mux2/1
  cos/1 -> Mux/4, Mux2/2
  Fcn/1 -> Mux1/1
  Fcn1/1 -> Mux1/2
  Mux1/1 -> ud1,uq1/1
  the/1 -> sin/1, cos/1
  Mux2/1 -> s1,c1/1

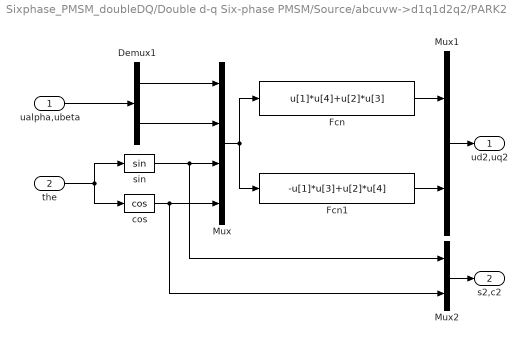
== system Sixphase_PMSM_doubleDQ/Double d-q Six-phase PMSM/Source/abcuvw->d1q1d2q2/PARK2 ==
  ualpha,ubeta : Inport
  the : Inport  Port=2
  Demux1 : Demux  Outputs=2
  Fcn : Fcn  Expr=u[1]*u[4]+u[2]*u[3]
  Fcn1 : Fcn  Expr=-u[1]*u[3]+u[2]*u[4]
  Mux : Mux
  Mux1 : Mux  Inputs=2
  Mux2 : Mux  Inputs=2
  cos : Trigonometry  Operator=cos
  sin : Trigonometry
  ud2,uq2 : Outport
  s2,c2 : Outport  Port=2
  wires:
  Mux/1 -> Fcn/1, Fcn1/1
  ualpha,ubeta/1 -> Demux1/1
  Demux1/1 -> Mux/1
  Demux1/2 -> Mux/2
  sin/1 -> Mux/3, Mux2/1
  cos/1 -> Mux/4, Mux2/2
  Fcn/1 -> Mux1/1
  Fcn1/1 -> Mux1/2
  Mux1/1 -> ud2,uq2/1
  the/1 -> sin/1, cos/1
  Mux2/1 -> s2,c2/1

== system Sixphase_PMSM_doubleDQ/Double d-q Six-phase PMSM/Source/d1q1d2q2->abcuvw/ICLARKE1 ==
  ialpha1.ibeta1 : Inport
  Fcn : Fcn  Expr=u[1]
  Fcn1 : Fcn  Expr=-1/2*u[1]+sqrt(3)/2*u[2]
  Fcn2 : Fcn  Expr=-1/2*u[1]-sqrt(3)/2*u[2]
  Mux : Mux  Inputs=3
  iabc : Outport
  wires:
  ialpha1.ibeta1/1 -> Fcn/1, Fcn1/1, Fcn2/1
  Fcn/1 -> Mux/1
  Fcn1/1 -> Mux/2
  Fcn2/1 -> Mux/3
  Mux/1 -> iabc/1

== system Sixphase_PMSM_doubleDQ/Double d-q Six-phase PMSM/Source/d1q1d2q2->abcuvw/ICLARKE2 ==
  ialpha2.ibeta2 : Inport
  Fcn : Fcn  Expr=u[1]
  Fcn1 : Fcn  Expr=-1/2*u[1]+sqrt(3)/2*u[2]
  Fcn2 : Fcn  Expr=-1/2*u[1]-sqrt(3)/2*u[2]
  Mux : Mux  Inputs=3
  ixyz : Outport
  wires:
  ialpha2.ibeta2/1 -> Fcn/1, Fcn1/1, Fcn2/1
  Fcn/1 -> Mux/1
  Fcn1/1 -> Mux/2
  Fcn2/1 -> Mux/3
  Mux/1 -> ixyz/1

== system Sixphase_PMSM_doubleDQ/Double d-q Six-phase PMSM/Source/d1q1d2q2->abcuvw/IPARK ==
  id1,iq1 : Inport
  s1,c1 : Inport  Port=2
  Demux : Demux  Outputs=2
  Demux1 : Demux  Outputs=2
  Fcn : Fcn  Expr=u[1]*u[4]-u[2]*u[3]
  Fcn1 : Fcn  Expr=u[1]*u[3]+u[2]*u[4]
  Mux : Mux
  Mux1 : Mux  Inputs=2
  ialpha1,ibeta1 : Outport
  wires:
  Mux/1 -> Fcn1/1, Fcn/1
  id1,iq1/1 -> Demux/1
  Demux/1 -> Mux/1
  Demux/2 -> Mux/2
  Demux1/1 -> Mux/3
  Demux1/2 -> Mux/4
  s1,c1/1 -> Demux1/1
  Fcn1/1 -> Mux1/2
  Fcn/1 -> Mux1/1
  Mux1/1 -> ialpha1,ibeta1/1

== system Sixphase_PMSM_doubleDQ/Double d-q Six-phase PMSM/Source/d1q1d2q2->abcuvw/IPARK1 ==
  id2,iq2 : Inport
  s2,c2 : Inport  Port=2
  Demux : Demux  Outputs=2
  Demux1 : Demux  Outputs=2
  Fcn : Fcn  Expr=u[1]*u[4]-u[2]*u[3]
  Fcn1 : Fcn  Expr=u[1]*u[3]+u[2]*u[4]
  Mux : Mux
  Mux1 : Mux  Inputs=2
  ialpha2,ibeta2 : Outport
  wires:
  Mux/1 -> Fcn1/1, Fcn/1
  id2,iq2/1 -> Demux/1
  Demux/1 -> Mux/1
  Demux/2 -> Mux/2
  Demux1/1 -> Mux/3
  Demux1/2 -> Mux/4
  s2,c2/1 -> Demux1/1
  Fcn1/1 -> Mux1/2
  Fcn/1 -> Mux1/1
  Mux1/1 -> ialpha2,ibeta2/1
